simulink model "function_to_block"  (R2018a)
settings: Solver=VariableStepAuto  StartTime=0.0  StopTime=10.0  RelTol=1e-3
settings Model: Creator=root  LastModifiedBy=root

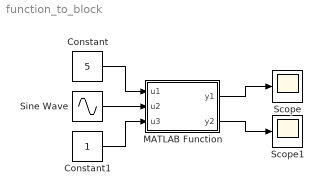
== system function_to_block ==
  Constant : Constant  Value=5
  Constant1 : Constant
  MATLAB Function : MATLAB Function  TreatAsAtomicUnit=on
  Scope : Scope
  Scope1 : Scope
  Sine Wave : Sin  SampleTime=0
  wires:
  Constant/1 -> MATLAB Function/1(u1)
  Sine Wave/1 -> MATLAB Function/2(u2)
  Constant1/1 -> MATLAB Function/3(u3)
  MATLAB Function/1(y1) -> Scope/1
  MATLAB Function/2(y2) -> Scope1/1

== matlab function function_to_block/MATLAB Function ==
  data: u1 input; y1 output; u2 input; u3 input; y2 output
function [y1,y2] = exemple(u1,u2,u3)

y1= u1+u2;
y2= u2+u3;
